simulink model "randomball"  (R2016a)
settings: Solver=FixedStepDiscrete  StartTime=0.0  StopTime=10.0  FixedStep=0.1  RelTol=1e-3
settings Model: Creator=areej_ofamech  LastModifiedBy=areej_ofamech
settings SolverCC: AutoInsertRateTranBlk=on
settings DataIOCC: LimitDataPoints=on
settings DebuggingCC: AllowSymbolicDim=off
settings ConfigComp: CovModelRefEnable=Off  CovSFcnEnable=off

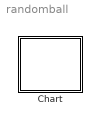
== system randomball ==
  Chart : Stateflow chart  TreatAsAtomicUnit=on

== stateflow chart randomball/Chart ==
  state b
    entry: x=uint8(2*rand(1));
  state a
    entry: x=uint8(2*rand(1));
  state c
    entry: x=uint8(2*rand(1));
  state d
    entry: x=uint8(2*rand(1));
  (default) -> b
  a -> b [order 1] : [x==1]
  b -> a [order 1] : [x==1]
  d -> b [order 3] : [x==0]
  c -> b [order 3] : [x==0]
  b -> d [order 2] : [x==2]
  d -> b [order 2] : [x==2]
  b -> d [order 3] : [x==0]
  c -> b [order 1] : [x==1]
  a -> c [order 3] : [x==0]
  c -> a [order 2] : [x==2]
  d -> c [order 1] : [x==1]
  a -> d [order 2] : [x==2]
  data: x local
